simulink model "Module4_No3"  (R2021b)
settings: Solver=VariableStepAuto  StartTime=0.0  StopTime=10.0  RelTol=1e-3
settings Model: Creator=Lenovo  LastModifiedBy=Lenovo

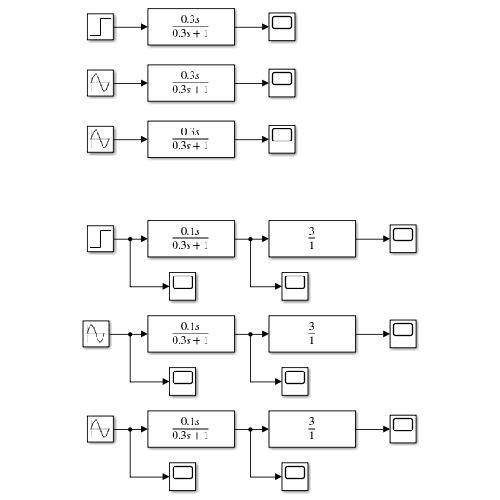
[thumbnail: Simulink's stored preview of the top-level diagram]
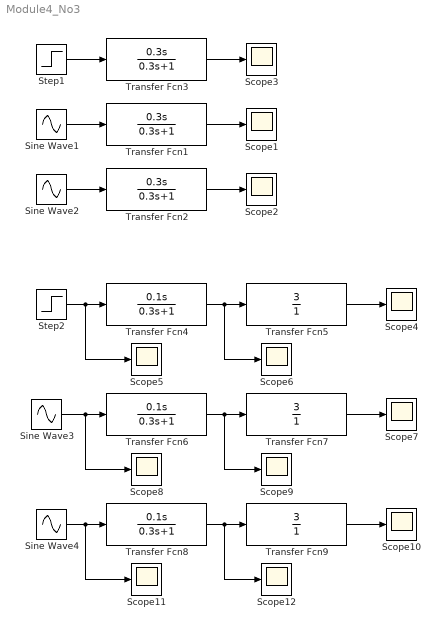
== system Module4_No3 ==
  Scope{1..12} (12 alike) : Scope
  Sine Wave1 : Sin  Amplitude=0.1  Bias=10  Frequency=20*pi  SampleTime=0
  Sine Wave2 : Sin  Amplitude=0.1  Bias=10  Frequency=0.2*pi  SampleTime=0
  Sine Wave3 : Sin  Amplitude=0.1  Bias=10  Frequency=20*pi  SampleTime=0
  Sine Wave4 : Sin  Amplitude=0.1  Bias=10  Frequency=0.2*pi  SampleTime=0
  Step1 : Step  Time=0  SampleTime=0
  Step2 : Step  Time=0  SampleTime=0
  Transfer Fcn1 : TransferFcn  Numerator=[0 0.3 0]  Denominator=[0 0.3 1]
  Transfer Fcn2 : TransferFcn  Numerator=[0 0.3 0]  Denominator=[0 0.3 1]
  Transfer Fcn3 : TransferFcn  Numerator=[0 0.3 0]  Denominator=[0 0.3 1]
  Transfer Fcn4 : TransferFcn  Numerator=[0 0.1 0]  Denominator=[0 0.3 1]
  Transfer Fcn5 : TransferFcn  Numerator=[0 0 3]  Denominator=[0 0 1]
  Transfer Fcn6 : TransferFcn  Numerator=[0 0.1 0]  Denominator=[0 0.3 1]
  Transfer Fcn7 : TransferFcn  Numerator=[0 0 3]  Denominator=[0 0 1]
  Transfer Fcn8 : TransferFcn  Numerator=[0 0.1 0]  Denominator=[0 0.3 1]
  Transfer Fcn9 : TransferFcn  Numerator=[0 0 3]  Denominator=[0 0 1]
  wires:
  Step1/1 -> Transfer Fcn3/1
  Transfer Fcn3/1 -> Scope3/1
  Transfer Fcn1/1 -> Scope1/1
  Sine Wave1/1 -> Transfer Fcn1/1
  Sine Wave2/1 -> Transfer Fcn2/1
  Transfer Fcn2/1 -> Scope2/1
  Step2/1 -> Scope5/1, Transfer Fcn4/1
  Transfer Fcn4/1 -> Scope6/1, Transfer Fcn5/1
  Transfer Fcn5/1 -> Scope4/1
  Sine Wave3/1 -> Scope8/1, Transfer Fcn6/1
  Transfer Fcn6/1 -> Scope9/1, Transfer Fcn7/1
  Transfer Fcn7/1 -> Scope7/1
  Transfer Fcn8/1 -> Scope12/1, Transfer Fcn9/1
  Transfer Fcn9/1 -> Scope10/1
  Sine Wave4/1 -> Scope11/1, Transfer Fcn8/1
